simulink model "Sensors"  (R2023b)
settings: Solver=FixedStepAuto  StartTime=0.0  StopTime=10.0  RelTol=1e-3
settings Model: Creator=cspt  LastModifiedBy=joser
settings SolverCC: AlgebraicLoopSolver=TrustRegion
settings DataIOCC: SaveOutput=off  ReturnWorkspaceOutputs=off
settings OptimizationCC: DefaultParameterBehavior=Inlined
settings DebuggingCC: UnconnectedInputMsg=warning  UnconnectedOutputMsg=warning  UnconnectedLineMsg=warning  ArithmeticOperatorsInVariantConditions=warning
settings ModelReferenceCC: EnableRefExpFcnMdlSchedulingChecks=on
settings SFSimCC: SimUseLocalCustomCode=off  CustomCodeUndefinedFunction=UseInterfaceOnly
settings RTWCC: Description=INTECRIO Real-Time Target  SystemTargetFile=irt.tlc  TemplateMakefile=irt_default_tmf  RTWUseLocalCustomCode=off
settings STFCustomTargetCC: UtilityFuncGeneration=Shared location  MatFileLogging=on  GRTInterface=on  SystemTargetFile=irt.tlc
settings GRTTargetCC: UtilityFuncGeneration=Shared location  ParMdlRefBuildCompliant=off  CompOptLevelCompliant=off  ConcurrentExecutionCompliant=off  CombineOutputUpdateFcns=off  CPPClassGenCompliant=off  GRTInterface=on  UseToolchainInfoCompliant=off  GenerateASAP2=on

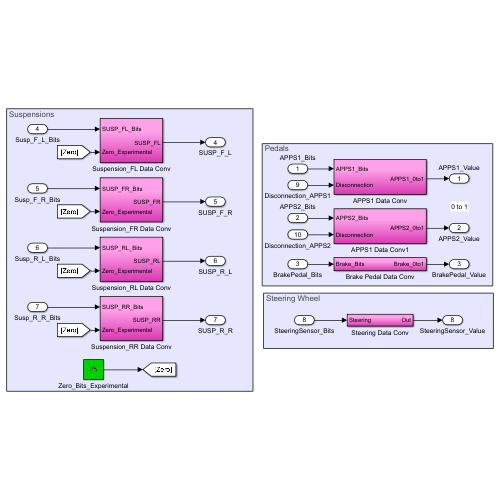
[thumbnail: Simulink's stored preview of the top-level diagram]
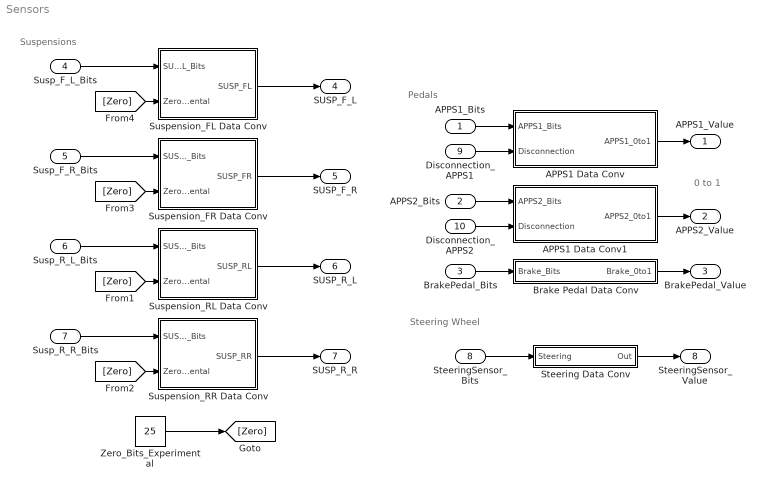
== system Sensors ==
  note: 0 to 1
  note: Pedals
  note: Suspensions
  note: Steering Wheel
  APPS1_Bits : Inport
  APPS2_Bits : Inport  Port=2
  BrakePedal_Bits : Inport  Port=3
  Susp_F_L_Bits : Inport  Port=4
  Susp_F_R_Bits : Inport  Port=5
  Susp_R_L_Bits : Inport  Port=6
  Susp_R_R_Bits : Inport  Port=7
  SteeringSensor_Bits : Inport  Port=8
  Disconnection_APPS1 : Inport  Port=9
  Disconnection_APPS2 : Inport  Port=10
  APPS1 Data Conv : Subsystem
  APPS1 Data Conv1 : Subsystem
  Brake Pedal Data Conv : Subsystem
  Steering Data Conv : Subsystem
  Suspension_FL Data Conv : Subsystem
  Suspension_FR Data Conv : Subsystem
  Suspension_RL Data Conv : Subsystem
  Suspension_RR Data Conv : Subsystem
  Zero_Bits_Experimental : Constant  Value=25
  APPS1_Value : Outport  VectorParamsAs1DForOutWhenUnconnected=off
  APPS2_Value : Outport  Port=2  VectorParamsAs1DForOutWhenUnconnected=off
  BrakePedal_Value : Outport  Port=3  VectorParamsAs1DForOutWhenUnconnected=off
  SUSP_F_L : Outport  Port=4  VectorParamsAs1DForOutWhenUnconnected=off
  SUSP_F_R : Outport  Port=5  VectorParamsAs1DForOutWhenUnconnected=off
  SUSP_R_L : Outport  Port=6  VectorParamsAs1DForOutWhenUnconnected=off
  SUSP_R_R : Outport  Port=7  VectorParamsAs1DForOutWhenUnconnected=off
  SteeringSensor_Value : Outport  Port=8  VectorParamsAs1DForOutWhenUnconnected=off
  wires:
  APPS1 Data Conv/1(APPS1_0to1) -> APPS1_Value/1
  APPS1_Bits/1 -> APPS1 Data Conv/1(APPS1_Bits)
  BrakePedal_Bits/1 -> Brake Pedal Data Conv/1(Brake_Bits)
  APPS1 Data Conv1/1(APPS2_0to1) -> APPS2_Value/1
  APPS2_Bits/1 -> APPS1 Data Conv1/1(APPS2_Bits)
  Susp_F_R_Bits/1 -> Suspension_FR Data Conv/1(SUSP_FR_Bits)
  Susp_R_R_Bits/1 -> Suspension_RR Data Conv/1(SUSP_RR_Bits)
  Susp_R_L_Bits/1 -> Suspension_RL Data Conv/1(SUSP_RL_Bits)
  Susp_F_L_Bits/1 -> Suspension_FL Data Conv/1(SUSP_FL_Bits)
  Suspension_RR Data Conv/1(SUSP_RR) -> SUSP_R_R/1
  Suspension_FR Data Conv/1(SUSP_FR) -> SUSP_F_R/1
  Suspension_RL Data Conv/1(SUSP_RL) -> SUSP_R_L/1
  SteeringSensor_Bits/1 -> Steering Data Conv/1("Steering ")
  Steering Data Conv/1(Out) -> SteeringSensor_Value/1
  Brake Pedal Data Conv/1(Brake_0to1) -> BrakePedal_Value/1
  Zero_Bits_Experimental/1 -> [Zero]
  [Zero] -> Suspension_RL Data Conv/2(Zero_Experimental)
  Suspension_FL Data Conv/1(SUSP_FL) -> SUSP_F_L/1
  [Zero] -> Suspension_RR Data Conv/2(Zero_Experimental)
  [Zero] -> Suspension_FR Data Conv/2(Zero_Experimental)
  [Zero] -> Suspension_FL Data Conv/2(Zero_Experimental)
  Disconnection_APPS1/1 -> APPS1 Data Conv/2(Disconnection)
  Disconnection_APPS2/1 -> APPS1 Data Conv1/2(Disconnection)

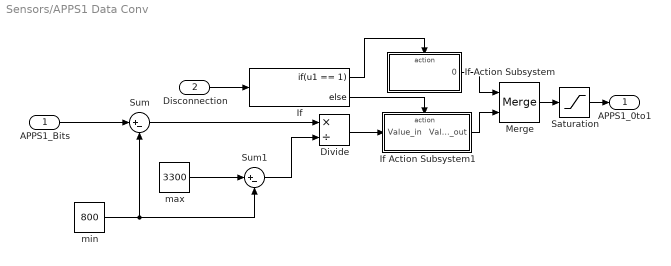
== system Sensors/APPS1 Data Conv ==
  APPS1_Bits : Inport
  Disconnection : Inport  Port=2
  Divide : Product  Inputs=*/
  If : If  IfExpression=u1 == 1
  If Action Subsystem : Subsystem  TreatAsAtomicUnit=on
  If Action Subsystem1 : Subsystem  TreatAsAtomicUnit=on
  Merge : Merge
  Saturation : Saturate  UpperLimit=1  LowerLimit=0
  Sum : Sum  Inputs=|+-
  Sum1 : Sum  Inputs=|+-
  max : Constant  Value=3300
  min : Constant  Value=800
  APPS1_0to1 : Outport  VectorParamsAs1DForOutWhenUnconnected=off
  wires:
  APPS1_Bits/1 -> Sum/1
  min/1 -> Sum/2, Sum1/2
  max/1 -> Sum1/1
  Sum/1 -> Divide/1
  Sum1/1 -> Divide/2
  Disconnection/1 -> If/1
  Merge/1 -> Saturation/1
  If/1 -> If Action Subsystem/Action
  If Action Subsystem/1(0) -> Merge/1
  If/2 -> If Action Subsystem1/Action
  Divide/1 -> If Action Subsystem1/1(Value_in)
  If Action Subsystem1/1(Value_out) -> Merge/2
  Saturation/1 -> APPS1_0to1/1

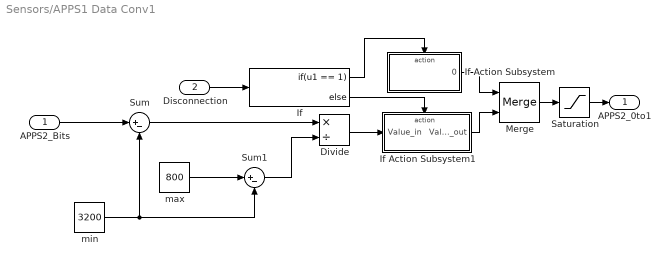
== system Sensors/APPS1 Data Conv1 ==
  APPS2_Bits : Inport
  Disconnection : Inport  Port=2
  Divide : Product  Inputs=*/
  If : If  IfExpression=u1 == 1
  If Action Subsystem : Subsystem  TreatAsAtomicUnit=on
  If Action Subsystem1 : Subsystem  TreatAsAtomicUnit=on
  Merge : Merge
  Saturation : Saturate  UpperLimit=1  LowerLimit=0
  Sum : Sum  Inputs=|+-
  Sum1 : Sum  Inputs=|+-
  max : Constant  Value=800
  min : Constant  Value=3200
  APPS2_0to1 : Outport  VectorParamsAs1DForOutWhenUnconnected=off
  wires:
  APPS2_Bits/1 -> Sum/1
  min/1 -> Sum/2, Sum1/2
  max/1 -> Sum1/1
  Sum/1 -> Divide/1
  Sum1/1 -> Divide/2
  Disconnection/1 -> If/1
  If/1 -> If Action Subsystem/Action
  If Action Subsystem/1(0) -> Merge/1
  If/2 -> If Action Subsystem1/Action
  Divide/1 -> If Action Subsystem1/1(Value_in)
  If Action Subsystem1/1(Value_out) -> Merge/2
  Merge/1 -> Saturation/1
  Saturation/1 -> APPS2_0to1/1

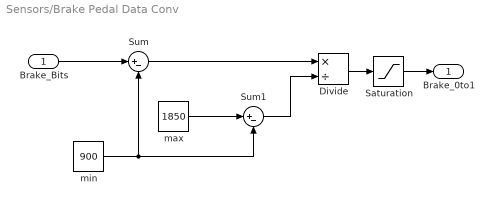
== system Sensors/Brake Pedal Data Conv ==
  Brake_Bits : Inport
  Divide : Product  Inputs=*/
  Saturation : Saturate  UpperLimit=1  LowerLimit=0
  Sum : Sum  Inputs=|+-
  Sum1 : Sum  Inputs=|+-
  max : Constant  Value=1850
  min : Constant  Value=900
  Brake_0to1 : Outport  VectorParamsAs1DForOutWhenUnconnected=off
  wires:
  Sum1/1 -> Divide/2
  Sum/1 -> Divide/1
  Divide/1 -> Saturation/1
  max/1 -> Sum1/1
  Brake_Bits/1 -> Sum/1
  min/1 -> Sum/2, Sum1/2
  Saturation/1 -> Brake_0to1/1

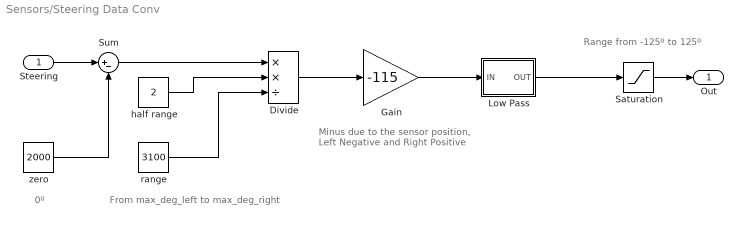
== system Sensors/Steering Data Conv ==
  note: Range from -125º to 125º
  note: From max_deg_left to max_deg_right
  note: 0º
  note: Minus due to the sensor position,
      | Left Negative and Right Positive
  "Steering " : Inport
  Divide : Product  Inputs=**/
  Gain : Gain  Gain=-115
  Low Pass : Subsystem  TreatAsAtomicUnit=on
  Saturation : Saturate  UpperLimit=125  LowerLimit=-125
  Sum : Sum  Inputs=|+-
  half range : Constant  Value=2
  range : Constant  Value=3100
  zero : Constant  Value=2000
  Out : Outport  VectorParamsAs1DForOutWhenUnconnected=off
  wires:
  zero/1 -> Sum/2
  Sum/1 -> Divide/1
  Divide/1 -> Gain/1
  range/1 -> Divide/3
  half range/1 -> Divide/2
  "Steering "/1 -> Sum/1
  Gain/1 -> Low Pass/1(IN)
  Low Pass/1(OUT) -> Saturation/1
  Saturation/1 -> Out/1

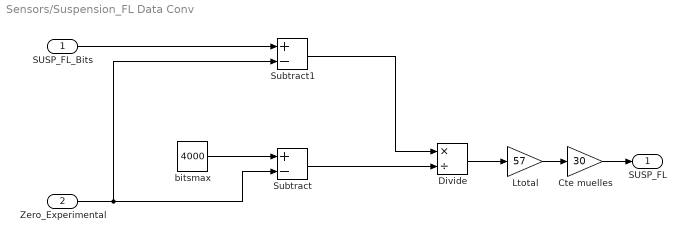
== system Sensors/Suspension_FL Data Conv ==
  SUSP_FL_Bits : Inport
  Zero_Experimental : Inport  Port=2
  Cte muelles : Gain  Gain=30
  Divide : Product  Inputs=*/
  Ltotal : Gain  Gain=57
  Subtract : Sum  Inputs=+-
  Subtract1 : Sum  Inputs=+-
  "bitsmax " : Constant  Value=4000
  SUSP_FL : Outport  VectorParamsAs1DForOutWhenUnconnected=off
  wires:
  Cte muelles/1 -> SUSP_FL/1
  Ltotal/1 -> Cte muelles/1
  Divide/1 -> Ltotal/1
  Zero_Experimental/1 -> Subtract1/2, Subtract/2
  Subtract1/1 -> Divide/1
  "bitsmax "/1 -> Subtract/1
  Subtract/1 -> Divide/2
  SUSP_FL_Bits/1 -> Subtract1/1

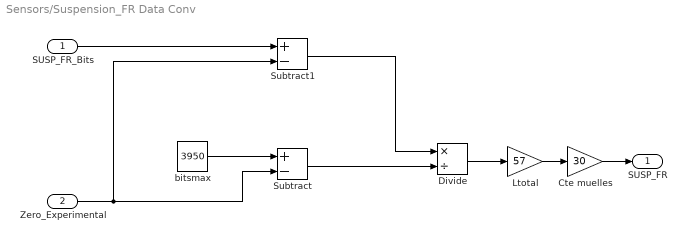
== system Sensors/Suspension_FR Data Conv ==
  SUSP_FR_Bits : Inport
  Zero_Experimental : Inport  Port=2
  Cte muelles : Gain  Gain=30
  Divide : Product  Inputs=*/
  Ltotal : Gain  Gain=57
  Subtract : Sum  Inputs=+-
  Subtract1 : Sum  Inputs=+-
  "bitsmax " : Constant  Value=3950
  SUSP_FR : Outport  VectorParamsAs1DForOutWhenUnconnected=off
  wires:
  Cte muelles/1 -> SUSP_FR/1
  Ltotal/1 -> Cte muelles/1
  Divide/1 -> Ltotal/1
  Zero_Experimental/1 -> Subtract1/2, Subtract/2
  Subtract1/1 -> Divide/1
  "bitsmax "/1 -> Subtract/1
  Subtract/1 -> Divide/2
  SUSP_FR_Bits/1 -> Subtract1/1

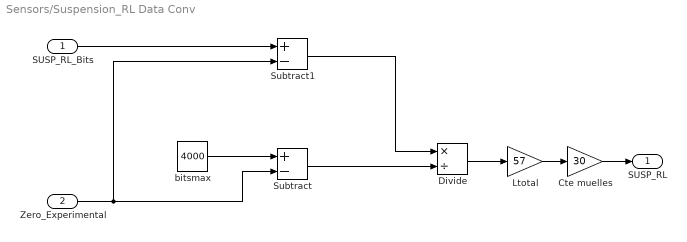
== system Sensors/Suspension_RL Data Conv ==
  SUSP_RL_Bits : Inport
  Zero_Experimental : Inport  Port=2
  Cte muelles : Gain  Gain=30
  Divide : Product  Inputs=*/
  Ltotal : Gain  Gain=57
  Subtract : Sum  Inputs=+-
  Subtract1 : Sum  Inputs=+-
  "bitsmax " : Constant  Value=4000
  SUSP_RL : Outport  VectorParamsAs1DForOutWhenUnconnected=off
  wires:
  Cte muelles/1 -> SUSP_RL/1
  Ltotal/1 -> Cte muelles/1
  Divide/1 -> Ltotal/1
  Zero_Experimental/1 -> Subtract1/2, Subtract/2
  Subtract1/1 -> Divide/1
  "bitsmax "/1 -> Subtract/1
  Subtract/1 -> Divide/2
  SUSP_RL_Bits/1 -> Subtract1/1

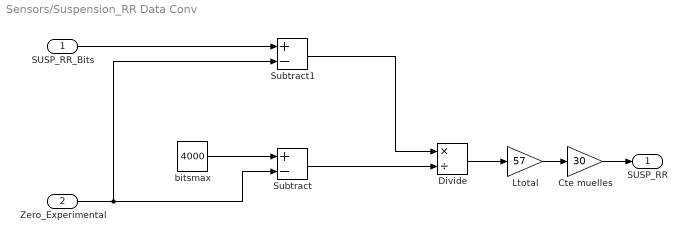
== system Sensors/Suspension_RR Data Conv ==
  SUSP_RR_Bits : Inport
  Zero_Experimental : Inport  Port=2
  Cte muelles : Gain  Gain=30
  Divide : Product  Inputs=*/
  Ltotal : Gain  Gain=57
  Subtract : Sum  Inputs=+-
  Subtract1 : Sum  Inputs=+-
  "bitsmax " : Constant  Value=4000
  SUSP_RR : Outport  VectorParamsAs1DForOutWhenUnconnected=off
  wires:
  Cte muelles/1 -> SUSP_RR/1
  Ltotal/1 -> Cte muelles/1
  Divide/1 -> Ltotal/1
  Zero_Experimental/1 -> Subtract1/2, Subtract/2
  Subtract1/1 -> Divide/1
  "bitsmax "/1 -> Subtract/1
  Subtract/1 -> Divide/2
  SUSP_RR_Bits/1 -> Subtract1/1

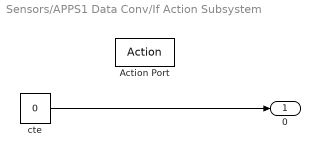
== system Sensors/APPS1 Data Conv/If Action Subsystem ==
  Action Port : ActionPort  ActionPortLabel=if(u1 == 1)
  cte : Constant  Value=0
  0 : Outport
  wires:
  cte/1 -> 0/1

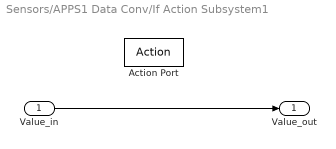
== system Sensors/APPS1 Data Conv/If Action Subsystem1 ==
  Value_in : Inport
  Action Port : ActionPort  ActionPortLabel=else
  Value_out : Outport
  wires:
  Value_in/1 -> Value_out/1

== system Sensors/APPS1 Data Conv1/If Action Subsystem ==
  Action Port : ActionPort  ActionPortLabel=if(u1 == 1)
  cte : Constant  Value=0
  0 : Outport
  wires:
  cte/1 -> 0/1

== system Sensors/APPS1 Data Conv1/If Action Subsystem1 ==
  Value_in : Inport
  Action Port : ActionPort  ActionPortLabel=else
  Value_out : Outport
  wires:
  Value_in/1 -> Value_out/1

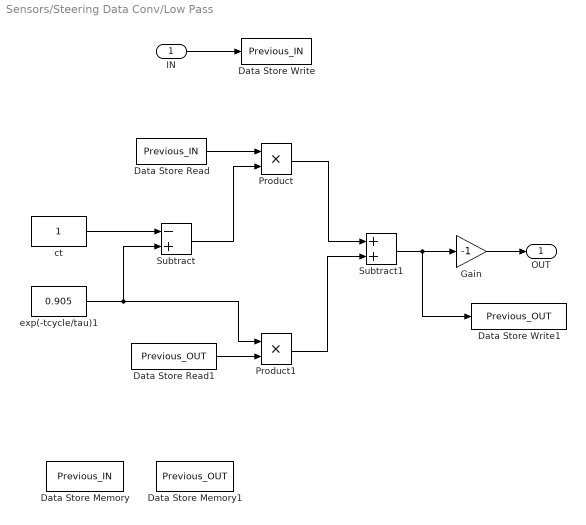
== system Sensors/Steering Data Conv/Low Pass ==
  IN : Inport
  Data Store Memory : DataStoreMemory  DataStoreName=Previous_IN  ReadBeforeWriteMsg=warning  WriteAfterWriteMsg=warning  WriteAfterReadMsg=warning  ShowAdditionalParam=off
  Data Store Memory1 : DataStoreMemory  DataStoreName=Previous_OUT  ReadBeforeWriteMsg=warning  WriteAfterWriteMsg=warning  WriteAfterReadMsg=warning  ShowAdditionalParam=off
  Data Store Read : DataStoreRead  DataStoreName=Previous_IN  IndexOptions=Index vector (dialog)  Indices=1  OutputSizes=1
  Data Store Read1 : DataStoreRead  DataStoreName=Previous_OUT  IndexOptions=Index vector (dialog)  Indices=1  OutputSizes=1
  Data Store Write : DataStoreWrite  DataStoreName=Previous_IN  IndexOptions=Index vector (dialog)  Indices=1  OutputSizes=1
  Data Store Write1 : DataStoreWrite  DataStoreName=Previous_OUT  IndexOptions=Index vector (dialog)  Indices=1  OutputSizes=1
  Gain : Gain  Gain=-1
  Product : Product
  Product1 : Product
  Subtract : Sum  Inputs=-+
  Subtract1 : Sum
  ct : Constant
  exp(-tcycle/tau)1 : Constant  Value=0.905
  OUT : Outport  VectorParamsAs1DForOutWhenUnconnected=off
  wires:
  IN/1 -> Data Store Write/1
  Data Store Read/1 -> Product/1
  Data Store Read1/1 -> Product1/2
  ct/1 -> Subtract/1
  Subtract/1 -> Product/2
  exp(-tcycle/tau)1/1 -> Product1/1, Subtract/2
  Product/1 -> Subtract1/1
  Product1/1 -> Subtract1/2
  Subtract1/1 -> Gain/1, Data Store Write1/1
  Gain/1 -> OUT/1
